simulink model "TestModel_HeliCE150_PID_FFCwithNN"  (R2020b)
settings: Solver=FixedStepAuto  StartTime=0.0  StopTime=Inf  FixedStep=1e-2  RelTol=1e-3
InitFcn:
  | Param_HeliCE150_PID_FFCwithNN
values from neighbouring files (symbols this model uses):
  a_1 = 0.105    [Main_HeliCE150_PID_FFCwithNN.m]    (also in Param_HeliCE150_PID_FFCwithNN.m)
  a_2 = 0.033    [Main_HeliCE150_PID_FFCwithNN.m]    (also in Param_HeliCE150_PID_FFCwithNN.m)
  b_1 = 0.00936    [Main_HeliCE150_PID_FFCwithNN.m]    (also in Param_HeliCE150_PID_FFCwithNN.m)
  b_2 = 0.0294    [Main_HeliCE150_PID_FFCwithNN.m]    (also in Param_HeliCE150_PID_FFCwithNN.m)
  B_phi = 0.00869    [Main_HeliCE150_PID_FFCwithNN.m]    (also in Param_HeliCE150_PID_FFCwithNN.m)
  B_psi = 0.00184    [Main_HeliCE150_PID_FFCwithNN.m]    (also in Param_HeliCE150_PID_FFCwithNN.m)
  I = 0.00437    [Main_HeliCE150_PID_FFCwithNN.m]    (also in Param_HeliCE150_PID_FFCwithNN.m)
  I_phi = 0.00414    [Main_HeliCE150_PID_FFCwithNN.m]    (also in Param_HeliCE150_PID_FFCwithNN.m)
  K_Gyro = 0.015    [Main_HeliCE150_PID_FFCwithNN.m]    (also in Param_HeliCE150_PID_FFCwithNN.m)
  K_r = 0.00162    [Main_HeliCE150_PID_FFCwithNN.m]    (also in Param_HeliCE150_PID_FFCwithNN.m)
  T_0r = 2.7    [Main_HeliCE150_PID_FFCwithNN.m]    (also in Param_HeliCE150_PID_FFCwithNN.m)
  T_1 = 0.3    [Main_HeliCE150_PID_FFCwithNN.m]    (also in Param_HeliCE150_PID_FFCwithNN.m)
  T_2 = 0.25    [Main_HeliCE150_PID_FFCwithNN.m]    (also in Param_HeliCE150_PID_FFCwithNN.m)
  T_pr = 0.75    [Main_HeliCE150_PID_FFCwithNN.m]    (also in Param_HeliCE150_PID_FFCwithNN.m)
  T_u1 = 0    [Main_HeliCE150_PID_FFCwithNN.m]    (also in Param_HeliCE150_PID_FFCwithNN.m)
  T_u2 = 1    [Main_HeliCE150_PID_FFCwithNN.m]    (also in Param_HeliCE150_PID_FFCwithNN.m)
  Tau_g = 0.0383    [Main_HeliCE150_PID_FFCwithNN.m]    (also in Param_HeliCE150_PID_FFCwithNN.m)
libraries: neural x24, pid_lib x3
(part 1 of 2)
settings Model: Creator=Juraj  LastModifiedBy=Juraj

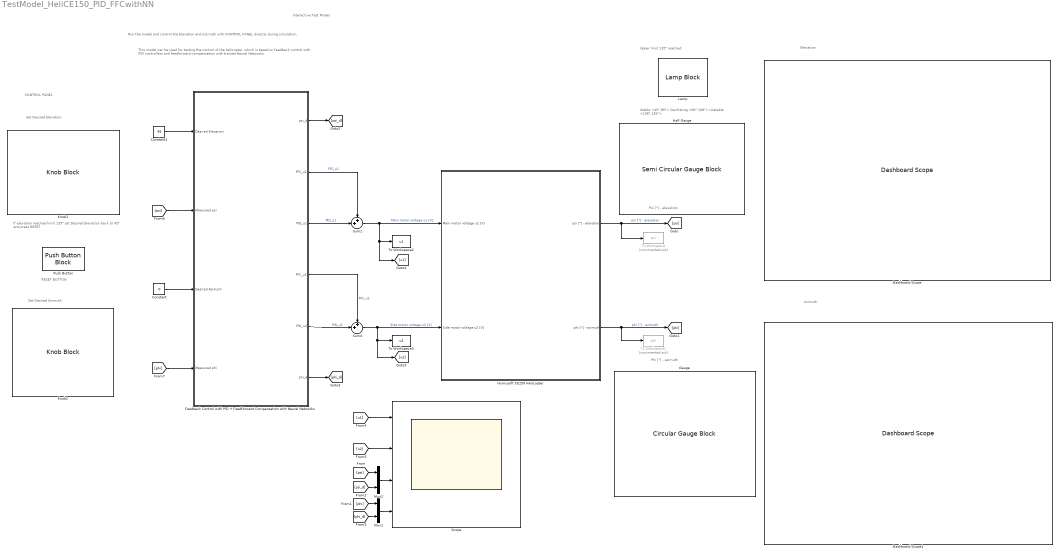
== system TestModel_HeliCE150_PID_FFCwithNN ==
  note: Stable <45°,90°>
      | Oscillating <90°,108°>
      | Unstable <108°,135°>
  note: Run the model and control the Elevation and Azimuth with CONTROL PANEL directly during simulation.
  note: Phi [°] - azimuth
  note: Psi [°] - elevation
  note: Elevation
  note: This model can be used for testing the control of the helicopter, which is based on
      | feedback control with PID controllers and feedforward compensation with trained Neural Networks
  note: Interactive Test Model
  note: CONTROL PANEL
  note: If elevation reached limit 135°
      | set Desired Elevation back to 45° and press RESET
  note: RESET BUTTON
  note: Set Desired Elevation
  note: Set Desired Azimuth
  note: Upper limit 135° reached
  note: Azimuth
  Constant : Constant  Value=0
  Constant1 : Constant  Value=45
  Dashboard Scope : DashboardScope  TimeSpan=1000  Ymin=40  Ymax=140  ScaleAtStop=off
  Dashboard Scope1 : DashboardScope  TimeSpan=1000  Ymin=-140  Ymax=140  ScaleAtStop=off
  Feedback Control with PID + Feedforward Compensation with Neural Networks : Subsystem
  Gauge : CircularGaugeBlock  LabelPosition=Hide  ScaleMin=-130  ScaleMax=130  TickInterval=20
  Half Gauge : SemiCircularGaugeBlock  LabelPosition=Hide  ScaleMin=45  ScaleMax=135  TickInterval=15
  Humusoft CE150 Helicopter : Subsystem
      mask Display: image('$imagefile'); % Use "Edit Image" on toolstrip to change.
  Knob1 : KnobBlock  LabelPosition=Hide  ScaleMin=45  ScaleMax=135  TickInterval=5
  Knob2 : KnobBlock  LabelPosition=Hide  ScaleMin=-130  ScaleMax=130  TickInterval=10
  Lamp : LampBlock  LabelPosition=Hide
  Mux1 : Mux  Inputs=2
  Mux2 : Mux  Inputs=2
  Push Button : PushButtonBlock  ButtonText=RESET
  Scope : Scope  NumInputPorts=4
  Sum1 : Sum  Inputs=++|
  Sum4 : Sum  Inputs=++|
  To Workspace : ToWorkspace  Commented=on  VariableName=psi  SampleTime=-1
  To Workspace1 : ToWorkspace  Commented=on  VariableName=phi  SampleTime=-1
  To Workspace2 : ToWorkspace  VariableName=u1  SampleTime=-1
  To Workspace3 : ToWorkspace  VariableName=u2  SampleTime=-1
  wires:
  [psi] -> Mux2/1
  Sum4/1 -> [u2], To Workspace3/1, Humusoft CE150 Helicopter/2(Side motor voltage u2 [V])  "Side motor voltage u2 [V]"
  Humusoft CE150 Helicopter/1(psi [°] - elevation) -> To Workspace/1, [psi]  "psi [°] - elevation"
  [u1] -> Scope/1
  Humusoft CE150 Helicopter/2(phi [°] - azimuth) -> To Workspace1/1, [phi]  "phi [°] - azimuth"
  [phi] -> Mux1/1
  [psi_d] -> Mux2/2
  Mux1/1 -> Scope/4
  Mux2/1 -> Scope/3
  Sum1/1 -> [u1], To Workspace2/1, Humusoft CE150 Helicopter/1(Main motor voltage u1 [V])  "Main motor voltage u1 [V]"
  [u2] -> Scope/2
  [phi_d] -> Mux1/2
  Feedback Control with PID + Feedforward Compensation with Neural Networks/6(phi_d) -> [phi_d]
  Feedback Control with PID + Feedforward Compensation with Neural Networks/5(PID_u2) -> Sum4/2  "PID_u2"
  Feedback Control with PID + Feedforward Compensation with Neural Networks/2(FFC_u1) -> Sum1/1  "FFC_u1"
  Feedback Control with PID + Feedforward Compensation with Neural Networks/1(psi_d) -> [psi_d]
  [psi] -> Feedback Control with PID + Feedforward Compensation with Neural Networks/2(Measured psi)
  Feedback Control with PID + Feedforward Compensation with Neural Networks/4(FFC_u2) -> Sum4/1  "FFC_u2"
  Feedback Control with PID + Feedforward Compensation with Neural Networks/3(PID_u1) -> Sum1/2  "PID_u1"
  [phi] -> Feedback Control with PID + Feedforward Compensation with Neural Networks/4(Measured phi)
  Constant/1 -> Feedback Control with PID + Feedforward Compensation with Neural Networks/3(Desired Azimuth)
  Constant1/1 -> Feedback Control with PID + Feedforward Compensation with Neural Networks/1(Desired Elevation)

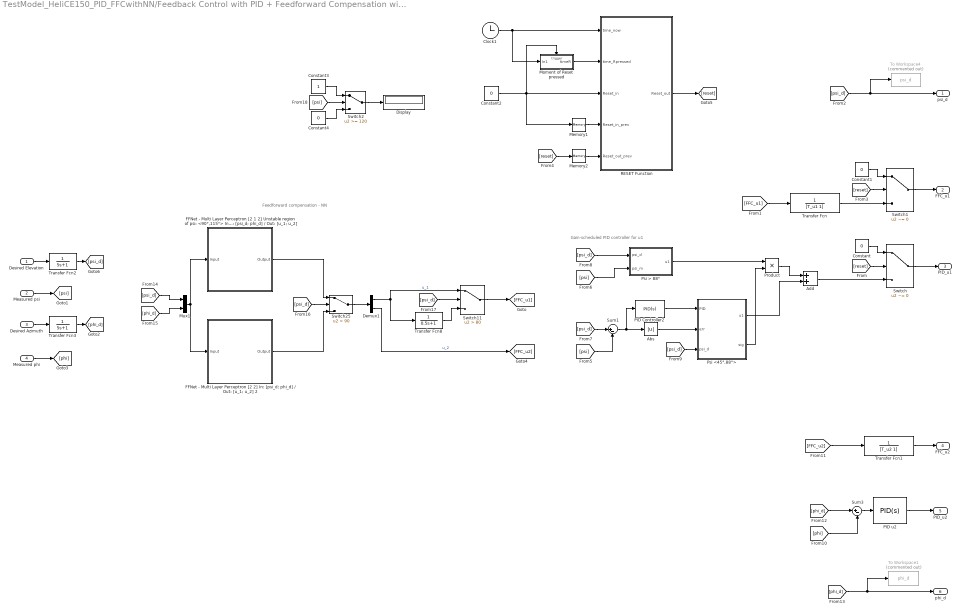
== system TestModel_HeliCE150_PID_FFCwithNN/Feedback Control with PID + Feedforward Compensation with Neural Networks ==
  note: Feedforward compensation - NN
  note: Gain-scheduled PID controller for u1
  Desired Elevation : Inport
  Measured psi : Inport  Port=2
  Desired Azimuth : Inport  Port=3
  Measured phi : Inport  Port=4
  Abs : Abs
  Add : Sum
  Clock1 : Clock
  Constant{,1..2,4} (4 alike) : Constant  Value=0
  Constant3 : Constant
  Demux1 : Demux  Outputs=2
  Display : Display
  FFNet - Multi Layer Perceptron [2 1 2] Unstable region of psi: <90°,115°> In: [psi_d; phi_d] / Out: [u_1; u_2] : Subsystem
      mask help: Feed-Forward Neural Network
      mask Display: e = 0.06;c1 = [120 150 230]/255;c2 = ([120 150 230]+0)/383;c3 = ([120 150 230]+128)/383;patch([0 1 1 0],[0 0 1 1],c1);patch([0 1 1 1-e 1-e 0+e],[0 0 1 1-e 0+e 0+e],c2);patch([0 0 1 1-e 0+e 0+e],[0 1 1 1-e 1-e 0+e],c3);plot([0 1 1 0 0],[0 0 1 1 0]);fprintf('NNET');port_label('input',1,' Input');port_label('output',1,'Output ');
  FFNet - Multi Layer Perceptron [2 2] In: [psi_d; phi_d] / Out: [u_1; u_2] 2 : Subsystem
      mask help: Feed-Forward Neural Network
      mask Display: e = 0.06;c1 = [120 150 230]/255;c2 = ([120 150 230]+0)/383;c3 = ([120 150 230]+128)/383;patch([0 1 1 0],[0 0 1 1],c1);patch([0 1 1 1-e 1-e 0+e],[0 0 1 1-e 0+e 0+e],c2);patch([0 0 1 1-e 0+e 0+e],[0 1 1 1-e 1-e 0+e],c3);plot([0 1 1 0 0],[0 0 1 1 0]);fprintf('NNET');port_label('input',1,' Input');port_label('output',1,'Output ');
  Memory1 : Memory
  Memory2 : Memory
  Moment of Reset pressed : Subsystem  TreatAsAtomicUnit=on
  Mux1 : Mux  Inputs=2
  PID Controller2 : pid_lib/PID Controller  Controller=PID  Form=Parallel  TimeDomain=Continuous-time  UseExternalTs=off  SampleTime=-1  IntegratorMethod=Forward Euler  FilterMethod=Forward Euler  ControllerParametersSource=internal  P=0.001  I=0  D=0.005  UseFilter=on  N=100  TunerSelectOption=Transfer Function Based (PID Tuner App)  InitialConditionSource=internal  InitialConditionForIntegrator=0  InitialConditionForFilter=0  DifferentiatorICPrevScaledInput=0  ExternalReset=none  TrackingMode=off  Kt=1  LimitOutput=on  SatLimitsSource=internal  UpperSaturationLimit=1  LowerSaturationLimit=-1  LinearizeAsGain=on  AntiWindupMode=clamping  Kb=1  POutMin=[]  POutMax=[]  IOutMin=[]  IOutMax=[]  DOutMin=[]  DOutMax=[]  NOutMin=[]  NOutMax=[]  SumOutMin=[]  SumOutMax=[]  SaturationOutMin=[]  SaturationOutMax=[]  PParamMin=[]  PParamMax=[]  IParamMin=[]  IParamMax=[]  DParamMin=[]  DParamMax=[]  NParamMin=[]  NParamMax=[]  KbParamMin=[]  KbParamMax=[]  KtParamMin=[]  KtParamMax=[]  KbOutMin=[]  KbOutMax=[]  KtOutMin=[]  KtOutMax=[]  IntegratorOutMin=[]  IntegratorOutMax=[]  FilterOutMin=[]  FilterOutMax=[]  SumI1OutMin=[]  SumI1OutMax=[]  SumI2OutMin=[]  SumI2OutMax=[]  SumI3OutMin=[]  SumI3OutMax=[]  SumI4OutMin=[]  SumI4OutMax=[]  SumDOutMin=[]  SumDOutMax=[]  DifferentiatorOutMin=[]  DifferentiatorOutMax=[]  FilterDiffOutCoefMin=[]  FilterDiffOutCoefMax=[]  ReciprocalOutMin=[]  ReciprocalOutMax=[]  SumDenOutMin=[]  SumDenOutMax=[]  SumNumOutMin=[]  SumNumOutMax=[]  DivideOutMin=[]  DivideOutMax=[]  UdiffTsProdOutMin=[]  UdiffTsProdOutMax=[]  NTsProdOutMin=[]  NTsProdOutMax=[]  UintegralTsProdOutMin=[]  UintegralTsProdOutMax=[]  UngainTsProdOutMin=[]  UngainTsProdOutMax=[]  IntegratorContinuousStateAttributes=''  IntegratorStateMustResolveToSignalObject=off  IntegratorRTWStateStorageClass=Auto  FilterContinuousStateAttributes=''  FilterStateMustResolveToSignalObject=off  FilterRTWStateStorageClass=Auto  ParallelPVariant=InternalParameters  IdealPVariant=Disabled  IVariant=InternalParameters  DVariant=InternalParameters  IntegratorVariant=Continuous  SatVariant=Enabled  AWVariant=ContClampingParallel  PCopyVariant=Disabled  TRVariant=Disabled  FdbkBlocksVariant=Forward  IdealPFdbkVariant=Disabled  SatFdbkVariant=Disabled  DerivativeFilterVariant=ContFilter  NVariant=InternalParameters  NCopyVariant=Disabled  FilterICVariant=InternalICsFilter  IntegratorICVariant=InternalICs  ExternalResetVariant=Disabled  TRSumVariant=Passthrough  SumFdbkVariant=Disabled  SumVariant=Sum_PID  TsampFilterVariant=InternalTs  TsampNgainVariant=Passthrough  TsampIntegralVariant=Passthrough  ExternalSaturationOutDataTypeStr=Inherit: Same as second input
  PID u2 : pid_lib/PID Controller  Controller=PID  Form=Parallel  TimeDomain=Continuous-time  UseExternalTs=off  SampleTime=-1  IntegratorMethod=Forward Euler  FilterMethod=Forward Euler  ControllerParametersSource=internal  P=0.01  I=0  D=0.01  UseFilter=on  N=100  TunerSelectOption=Transfer Function Based (PID Tuner App)  InitialConditionSource=internal  InitialConditionForIntegrator=0  InitialConditionForFilter=0  DifferentiatorICPrevScaledInput=0  ExternalReset=none  TrackingMode=off  Kt=1  LimitOutput=on  SatLimitsSource=internal  UpperSaturationLimit=1  LowerSaturationLimit=-1  LinearizeAsGain=on  AntiWindupMode=none  Kb=1  POutMin=[]  POutMax=[]  IOutMin=[]  IOutMax=[]  DOutMin=[]  DOutMax=[]  NOutMin=[]  NOutMax=[]  SumOutMin=[]  SumOutMax=[]  SaturationOutMin=[]  SaturationOutMax=[]  PParamMin=[]  PParamMax=[]  IParamMin=[]  IParamMax=[]  DParamMin=[]  DParamMax=[]  NParamMin=[]  NParamMax=[]  KbParamMin=[]  KbParamMax=[]  KtParamMin=[]  KtParamMax=[]  KbOutMin=[]  KbOutMax=[]  KtOutMin=[]  KtOutMax=[]  IntegratorOutMin=[]  IntegratorOutMax=[]  FilterOutMin=[]  FilterOutMax=[]  SumI1OutMin=[]  SumI1OutMax=[]  SumI2OutMin=[]  SumI2OutMax=[]  SumI3OutMin=[]  SumI3OutMax=[]  SumI4OutMin=[]  SumI4OutMax=[]  SumDOutMin=[]  SumDOutMax=[]  DifferentiatorOutMin=[]  DifferentiatorOutMax=[]  FilterDiffOutCoefMin=[]  FilterDiffOutCoefMax=[]  ReciprocalOutMin=[]  ReciprocalOutMax=[]  SumDenOutMin=[]  SumDenOutMax=[]  SumNumOutMin=[]  SumNumOutMax=[]  DivideOutMin=[]  DivideOutMax=[]  UdiffTsProdOutMin=[]  UdiffTsProdOutMax=[]  NTsProdOutMin=[]  NTsProdOutMax=[]  UintegralTsProdOutMin=[]  UintegralTsProdOutMax=[]  UngainTsProdOutMin=[]  UngainTsProdOutMax=[]  IntegratorContinuousStateAttributes=''  IntegratorStateMustResolveToSignalObject=off  IntegratorRTWStateStorageClass=Auto  FilterContinuousStateAttributes=''  FilterStateMustResolveToSignalObject=off  FilterRTWStateStorageClass=Auto  ParallelPVariant=InternalParameters  IdealPVariant=Disabled  IVariant=InternalParameters  DVariant=InternalParameters  IntegratorVariant=Continuous  SatVariant=Enabled  AWVariant=Passthrough  PCopyVariant=Disabled  TRVariant=Disabled  FdbkBlocksVariant=Forward  IdealPFdbkVariant=Disabled  SatFdbkVariant=Disabled  DerivativeFilterVariant=ContFilter  NVariant=InternalParameters  NCopyVariant=Disabled  FilterICVariant=InternalICsFilter  IntegratorICVariant=InternalICs  ExternalResetVariant=Disabled  TRSumVariant=Passthrough  SumFdbkVariant=Disabled  SumVariant=Sum_PID  TsampFilterVariant=InternalTs  TsampNgainVariant=Passthrough  TsampIntegralVariant=Passthrough  ExternalSaturationOutDataTypeStr=Inherit: Same as second input
  Product : Product
  Psi <45°,88°> : MATLAB Function  TreatAsAtomicUnit=on
  Psi > 88° : Subsystem
  RESET Function : MATLAB Function  TreatAsAtomicUnit=on
  Sum1 : Sum  Inputs=|+-
  Sum3 : Sum  Inputs=|+-
  Switch : Switch  Criteria=u2 ~= 0
  Switch1 : Switch  Criteria=u2 ~= 0
  Switch11 : Switch  Criteria=u2 > Threshold  Threshold=80
  Switch2 : Switch  Threshold=120
  Switch25 : Switch  Criteria=u2 > Threshold  Threshold=90
  To Workspace1 : ToWorkspace  Commented=on  VariableName=phi_d  SampleTime=-1
  To Workspace4 : ToWorkspace  Commented=on  VariableName=psi_d  SampleTime=-1
  Transfer Fcn : TransferFcn  Denominator=[T_u1 1]
  Transfer Fcn1 : TransferFcn  Denominator=[T_u2 1]
  Transfer Fcn2 : TransferFcn  Denominator=[5 1]
  Transfer Fcn3 : TransferFcn  Denominator=[5 1]
  Transfer Fcn8 : TransferFcn  Denominator=[0.5 1]
  psi_d : Outport
  FFC_u1 : Outport  Port=2
  PID_u1 : Outport  Port=3
  FFC_u2 : Outport  Port=4
  PID_u2 : Outport  Port=5
  phi_d : Outport  Port=6
  wires:
  Sum3/1 -> PID u2/1
  Transfer Fcn/1 -> Switch1/3
  [FFC_u1] -> Transfer Fcn/1
  [psi_d] -> To Workspace4/1, psi_d/1
  Measured psi/1 -> [psi]
  Measured phi/1 -> [phi]
  Add/1 -> Switch/3
  Product/1 -> Add/1
  Psi <45°,88°>/1(u1) -> Add/2
  [psi_d] -> Psi <45°,88°>/3(psi_d)
  PID Controller2/1 -> Psi <45°,88°>/1(PID)
  Psi <45°,88°>/2(sig) -> Product/2
  [psi] -> Psi > 88°/2(psi_m)
  Psi > 88°/1(u1) -> Product/1
  [psi_d] -> Psi > 88°/1(psi_d)
  Sum1/1 -> Abs/1, PID Controller2/1
  [psi_d] -> Sum1/1
  [psi] -> Sum1/2
  Abs/1 -> Psi <45°,88°>/2(err)
  [FFC_u2] -> Transfer Fcn1/1
  Transfer Fcn1/1 -> FFC_u2/1
  [phi_d] -> Sum3/1
  [phi] -> Sum3/2
  PID u2/1 -> PID_u2/1
  [phi_d] -> phi_d/1, To Workspace1/1
  [psi_d] -> Switch25/2
  FFNet - Multi Layer Perceptron [2 2] In: [psi_d; phi_d] / Out: [u_1; u_2] 2/1(Output) -> Switch25/3
  FFNet - Multi Layer Perceptron [2 1 2] Unstable region of psi: <90°,115°> In: [psi_d; phi_d] / Out: [u_1; u_2]/1(Output) -> Switch25/1
  Switch11/1 -> [FFC_u1]
  [phi_d] -> Mux1/2
  [psi_d] -> Mux1/1
  Demux1/1 -> Transfer Fcn8/1, Switch11/1  "u_1"
  Mux1/1 -> FFNet - Multi Layer Perceptron [2 2] In: [psi_d; phi_d] / Out: [u_1; u_2] 2/1(Input), FFNet - Multi Layer Perceptron [2 1 2] Unstable region of psi: <90°,115°> In: [psi_d; phi_d] / Out: [u_1; u_2]/1(Input)
  Transfer Fcn8/1 -> Switch11/3
  [psi_d] -> Switch11/2
  Switch25/1 -> Demux1/1
  Demux1/2 -> [FFC_u2]  "u_2"
  Desired Elevation/1 -> Transfer Fcn2/1
  Desired Azimuth/1 -> Transfer Fcn3/1
  Transfer Fcn2/1 -> [psi_d]
  Transfer Fcn3/1 -> [phi_d]
  [reset] -> Switch/2
  Switch/1 -> PID_u1/1
  Constant/1 -> Switch/1
  [reset] -> Switch1/2
  Constant1/1 -> Switch1/1
  Switch1/1 -> FFC_u1/1
  RESET Function/1(Reset_out) -> [reset]
  Memory1/1 -> RESET Function/4(Reset_in_prev)
  Clock1/1 -> Moment of Reset pressed/1(In1), RESET Function/1(time_now)
  Constant2/1 -> RESET Function/3(Reset_in), Memory1/1, Moment of Reset pressed/Trigger
  Moment of Reset pressed/1(timeR) -> RESET Function/2(time_Rpressed)
  Memory2/1 -> RESET Function/5(Reset_out_prev)
  [reset] -> Memory2/1
  [psi] -> Switch2/2
  Constant4/1 -> Switch2/3
  Constant3/1 -> Switch2/1
  Switch2/1 -> Display/1

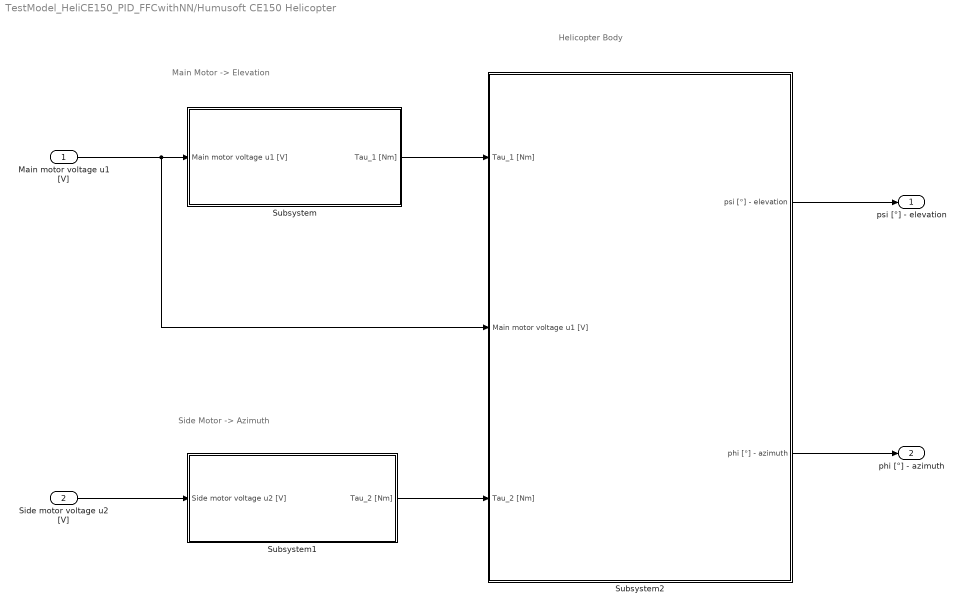
== system TestModel_HeliCE150_PID_FFCwithNN/Humusoft CE150 Helicopter ==
  note: Helicopter Body
  note: Side Motor -> Azimuth
  note: Main Motor -> Elevation
  Main motor voltage u1 [V] : Inport
  Side motor voltage u2 [V] : Inport  Port=2
  Subsystem : Subsystem
  Subsystem1 : Subsystem
  Subsystem2 : Subsystem
  psi [°] - elevation : Outport
  phi [°] - azimuth : Outport  Port=2
  wires:
  Main motor voltage u1 [V]/1 -> Subsystem2/2(Main motor voltage u1 [V]), Subsystem/1(Main motor voltage u1 [V])
  Side motor voltage u2 [V]/1 -> Subsystem1/1(Side motor voltage u2 [V])
  Subsystem/1(Tau_1 [Nm]) -> Subsystem2/1(Tau_1 [Nm])
  Subsystem1/1(Tau_2 [Nm]) -> Subsystem2/3(Tau_2 [Nm])
  Subsystem2/1(psi [°] - elevation) -> psi [°] - elevation/1
  Subsystem2/2(phi [°] - azimuth) -> phi [°] - azimuth/1

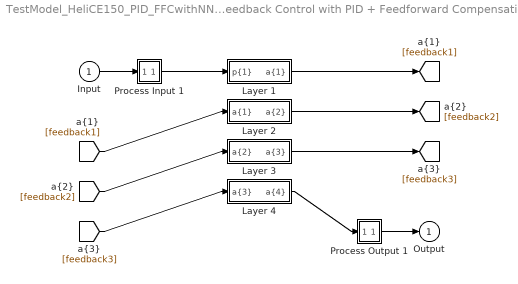
== system TestModel_HeliCE150_PID_FFCwithNN/Feedback Control with PID + Feedforward Compensation with Neural Networks/FFNet - Multi Layer Perceptron [2 1 2] Unstable region of psi: <90°,115°> In: [psi_d; phi_d] // Out: [u_1; u_2] ==
  Input : Inport  PortDimensions=2
      mask Display: e = 0.06;c1 = [120 230 180]/255;c2 = ([120 230 180]+0)/(256+128);c3 = ([120 230 180]+128)/(256+128);patch([0 1 1 0],[0 0 1 1],c1);patch([0 1 1 1-e 1-e 0+e],[0 0 1 1-e 0+e 0+e],c2);patch([0 0 1 1-e 0+e 0+e],[0 1 1 1-e 1-e 0+e],c3);plot([0 1 1 0 0],[0 0 1 1 0]);
  Layer 1 : Subsystem
      mask Display: e = 0.06;c1 = [120 150 230]/255;c2 = ([120 150 230]+0)/383;c3 = ([120 150 230]+128)/383;patch([0 1 1 0],[0 0 1 1],c1);patch([0 1 1 1-e 1-e 0+e],[0 0 1 1-e 0+e 0+e],c2);patch([0 0 1 1-e 0+e 0+e],[0 1 1 1-e 1-e 0+e],c3);plot([0 1 1 0 0],[0 0 1 1 0]);
  Layer 2 : Subsystem
      mask Display: e = 0.06;c1 = [120 150 230]/255;c2 = ([120 150 230]+0)/383;c3 = ([120 150 230]+128)/383;patch([0 1 1 0],[0 0 1 1],c1);patch([0 1 1 1-e 1-e 0+e],[0 0 1 1-e 0+e 0+e],c2);patch([0 0 1 1-e 0+e 0+e],[0 1 1 1-e 1-e 0+e],c3);plot([0 1 1 0 0],[0 0 1 1 0]);
  Layer 3 : Subsystem
      mask Display: e = 0.06;c1 = [120 150 230]/255;c2 = ([120 150 230]+0)/383;c3 = ([120 150 230]+128)/383;patch([0 1 1 0],[0 0 1 1],c1);patch([0 1 1 1-e 1-e 0+e],[0 0 1 1-e 0+e 0+e],c2);patch([0 0 1 1-e 0+e 0+e],[0 1 1 1-e 1-e 0+e],c3);plot([0 1 1 0 0],[0 0 1 1 0]);
  Layer 4 : Subsystem
      mask Display: e = 0.06;c1 = [120 150 230]/255;c2 = ([120 150 230]+0)/383;c3 = ([120 150 230]+128)/383;patch([0 1 1 0],[0 0 1 1],c1);patch([0 1 1 1-e 1-e 0+e],[0 0 1 1-e 0+e 0+e],c2);patch([0 0 1 1-e 0+e 0+e],[0 1 1 1-e 1-e 0+e],c3);plot([0 1 1 0 0],[0 0 1 1 0]);
  Process Input 1 : Subsystem
      mask Display: e = 0.06;c1 = [120 150 230]/255;c2 = ([120 150 230]+0)/383;c3 = ([120 150 230]+128)/383;patch([0 1 1 0],[0 0 1 1],c1);patch([0 1 1 1-e 1-e 0+e],[0 0 1 1-e 0+e 0+e],c2);patch([0 0 1 1-e 0+e 0+e],[0 1 1 1-e 1-e 0+e],c3);plot([0 1 1 0 0],[0 0 1 1 0]);
  Process Output 1 : Subsystem
      mask Display: e = 0.06;c1 = [120 150 230]/255;c2 = ([120 150 230]+0)/383;c3 = ([120 150 230]+128)/383;patch([0 1 1 0],[0 0 1 1],c1);patch([0 1 1 1-e 1-e 0+e],[0 0 1 1-e 0+e 0+e],c2);patch([0 0 1 1-e 0+e 0+e],[0 1 1 1-e 1-e 0+e],c3);plot([0 1 1 0 0],[0 0 1 1 0]);
  Output : Outport  InitialOutput=[0;0]
      mask Display: e = 0.06;c1 = [120 230 180]/255;c2 = ([120 230 180]+0)/(256+128);c3 = ([120 230 180]+128)/(256+128);patch([0 1 1 0],[0 0 1 1],c1);patch([0 1 1 1-e 1-e 0+e],[0 0 1 1-e 0+e 0+e],c2);patch([0 0 1 1-e 0+e 0+e],[0 1 1 1-e 1-e 0+e],c3);plot([0 1 1 0 0],[0 0 1 1 0]);
  wires:
  Input/1 -> Process Input 1/1(x)
  Process Output 1/1(y) -> Output/1
  Process Input 1/1(p) -> Layer 1/1("p{1}")
  Layer 1/1("a{1}") -> [feedback1]
  [feedback1] -> Layer 2/1("a{1} ")
  Layer 2/1("a{2}") -> [feedback2]
  [feedback2] -> Layer 3/1("a{2} ")
  Layer 3/1("a{3}") -> [feedback3]
  [feedback3] -> Layer 4/1("a{3} ")
  Layer 4/1("a{4}") -> Process Output 1/1(a)

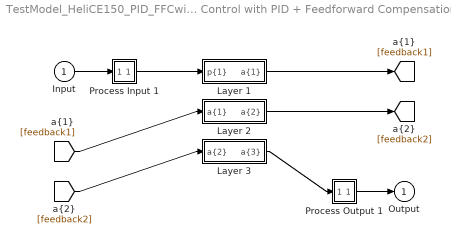
== system TestModel_HeliCE150_PID_FFCwithNN/Feedback Control with PID + Feedforward Compensation with Neural Networks/FFNet - Multi Layer Perceptron [2 2] In: [psi_d; phi_d] // Out: [u_1; u_2] 2 ==
  Input : Inport  PortDimensions=2
      mask Display: e = 0.06;c1 = [120 230 180]/255;c2 = ([120 230 180]+0)/(256+128);c3 = ([120 230 180]+128)/(256+128);patch([0 1 1 0],[0 0 1 1],c1);patch([0 1 1 1-e 1-e 0+e],[0 0 1 1-e 0+e 0+e],c2);patch([0 0 1 1-e 0+e 0+e],[0 1 1 1-e 1-e 0+e],c3);plot([0 1 1 0 0],[0 0 1 1 0]);
  Layer 1 : Subsystem
      mask Display: e = 0.06;c1 = [120 150 230]/255;c2 = ([120 150 230]+0)/383;c3 = ([120 150 230]+128)/383;patch([0 1 1 0],[0 0 1 1],c1);patch([0 1 1 1-e 1-e 0+e],[0 0 1 1-e 0+e 0+e],c2);patch([0 0 1 1-e 0+e 0+e],[0 1 1 1-e 1-e 0+e],c3);plot([0 1 1 0 0],[0 0 1 1 0]);
  Layer 2 : Subsystem
      mask Display: e = 0.06;c1 = [120 150 230]/255;c2 = ([120 150 230]+0)/383;c3 = ([120 150 230]+128)/383;patch([0 1 1 0],[0 0 1 1],c1);patch([0 1 1 1-e 1-e 0+e],[0 0 1 1-e 0+e 0+e],c2);patch([0 0 1 1-e 0+e 0+e],[0 1 1 1-e 1-e 0+e],c3);plot([0 1 1 0 0],[0 0 1 1 0]);
  Layer 3 : Subsystem
      mask Display: e = 0.06;c1 = [120 150 230]/255;c2 = ([120 150 230]+0)/383;c3 = ([120 150 230]+128)/383;patch([0 1 1 0],[0 0 1 1],c1);patch([0 1 1 1-e 1-e 0+e],[0 0 1 1-e 0+e 0+e],c2);patch([0 0 1 1-e 0+e 0+e],[0 1 1 1-e 1-e 0+e],c3);plot([0 1 1 0 0],[0 0 1 1 0]);
  Process Input 1 : Subsystem
      mask Display: e = 0.06;c1 = [120 150 230]/255;c2 = ([120 150 230]+0)/383;c3 = ([120 150 230]+128)/383;patch([0 1 1 0],[0 0 1 1],c1);patch([0 1 1 1-e 1-e 0+e],[0 0 1 1-e 0+e 0+e],c2);patch([0 0 1 1-e 0+e 0+e],[0 1 1 1-e 1-e 0+e],c3);plot([0 1 1 0 0],[0 0 1 1 0]);
  Process Output 1 : Subsystem
      mask Display: e = 0.06;c1 = [120 150 230]/255;c2 = ([120 150 230]+0)/383;c3 = ([120 150 230]+128)/383;patch([0 1 1 0],[0 0 1 1],c1);patch([0 1 1 1-e 1-e 0+e],[0 0 1 1-e 0+e 0+e],c2);patch([0 0 1 1-e 0+e 0+e],[0 1 1 1-e 1-e 0+e],c3);plot([0 1 1 0 0],[0 0 1 1 0]);
  Output : Outport  InitialOutput=[0;0]
      mask Display: e = 0.06;c1 = [120 230 180]/255;c2 = ([120 230 180]+0)/(256+128);c3 = ([120 230 180]+128)/(256+128);patch([0 1 1 0],[0 0 1 1],c1);patch([0 1 1 1-e 1-e 0+e],[0 0 1 1-e 0+e 0+e],c2);patch([0 0 1 1-e 0+e 0+e],[0 1 1 1-e 1-e 0+e],c3);plot([0 1 1 0 0],[0 0 1 1 0]);
  wires:
  Layer 3/1("a{3}") -> Process Output 1/1(a)
  [feedback2] -> Layer 3/1("a{2} ")
  Layer 2/1("a{2}") -> [feedback2]
  [feedback1] -> Layer 2/1("a{1} ")
  Layer 1/1("a{1}") -> [feedback1]
  Process Input 1/1(p) -> Layer 1/1("p{1}")
  Process Output 1/1(y) -> Output/1
  Input/1 -> Process Input 1/1(x)

== system TestModel_HeliCE150_PID_FFCwithNN/Feedback Control with PID + Feedforward Compensation with Neural Networks/Moment of Reset pressed ==
  In1 : Inport
  Trigger : TriggerPort  VariantControl=(inherit)
  timeR : Outport
  wires:
  In1/1 -> timeR/1

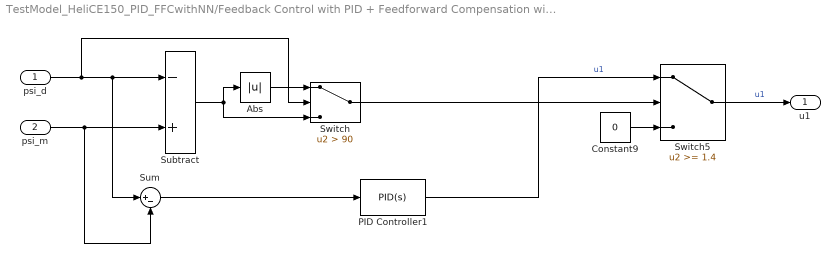
== system TestModel_HeliCE150_PID_FFCwithNN/Feedback Control with PID + Feedforward Compensation with Neural Networks/Psi > 88° ==
  psi_d : Inport
  psi_m : Inport  Port=2
  Abs : Abs
  Constant9 : Constant  Value=0
  PID Controller1 : pid_lib/PID Controller  Controller=PID  Form=Parallel  TimeDomain=Continuous-time  UseExternalTs=off  SampleTime=-1  IntegratorMethod=Forward Euler  FilterMethod=Forward Euler  ControllerParametersSource=internal  P=0.0001  I=0  D=0.015  UseFilter=on  N=100  TunerSelectOption=Transfer Function Based (PID Tuner App)  InitialConditionSource=internal  InitialConditionForIntegrator=0  InitialConditionForFilter=0  DifferentiatorICPrevScaledInput=0  ExternalReset=none  TrackingMode=off  Kt=1  LimitOutput=on  SatLimitsSource=internal  UpperSaturationLimit=1  LowerSaturationLimit=-1  LinearizeAsGain=on  AntiWindupMode=clamping  Kb=1  POutMin=[]  POutMax=[]  IOutMin=[]  IOutMax=[]  DOutMin=[]  DOutMax=[]  NOutMin=[]  NOutMax=[]  SumOutMin=[]  SumOutMax=[]  SaturationOutMin=[]  SaturationOutMax=[]  PParamMin=[]  PParamMax=[]  IParamMin=[]  IParamMax=[]  DParamMin=[]  DParamMax=[]  NParamMin=[]  NParamMax=[]  KbParamMin=[]  KbParamMax=[]  KtParamMin=[]  KtParamMax=[]  KbOutMin=[]  KbOutMax=[]  KtOutMin=[]  KtOutMax=[]  IntegratorOutMin=[]  IntegratorOutMax=[]  FilterOutMin=[]  FilterOutMax=[]  SumI1OutMin=[]  SumI1OutMax=[]  SumI2OutMin=[]  SumI2OutMax=[]  SumI3OutMin=[]  SumI3OutMax=[]  SumI4OutMin=[]  SumI4OutMax=[]  SumDOutMin=[]  SumDOutMax=[]  DifferentiatorOutMin=[]  DifferentiatorOutMax=[]  FilterDiffOutCoefMin=[]  FilterDiffOutCoefMax=[]  ReciprocalOutMin=[]  ReciprocalOutMax=[]  SumDenOutMin=[]  SumDenOutMax=[]  SumNumOutMin=[]  SumNumOutMax=[]  DivideOutMin=[]  DivideOutMax=[]  UdiffTsProdOutMin=[]  UdiffTsProdOutMax=[]  NTsProdOutMin=[]  NTsProdOutMax=[]  UintegralTsProdOutMin=[]  UintegralTsProdOutMax=[]  UngainTsProdOutMin=[]  UngainTsProdOutMax=[]  IntegratorContinuousStateAttributes=''  IntegratorStateMustResolveToSignalObject=off  IntegratorRTWStateStorageClass=Auto  FilterContinuousStateAttributes=''  FilterStateMustResolveToSignalObject=off  FilterRTWStateStorageClass=Auto  ParallelPVariant=InternalParameters  IdealPVariant=Disabled  IVariant=InternalParameters  DVariant=InternalParameters  IntegratorVariant=Continuous  SatVariant=Enabled  AWVariant=ContClampingParallel  PCopyVariant=Disabled  TRVariant=Disabled  FdbkBlocksVariant=Forward  IdealPFdbkVariant=Disabled  SatFdbkVariant=Disabled  DerivativeFilterVariant=ContFilter  NVariant=InternalParameters  NCopyVariant=Disabled  FilterICVariant=InternalICsFilter  IntegratorICVariant=InternalICs  ExternalResetVariant=Disabled  TRSumVariant=Passthrough  SumFdbkVariant=Disabled  SumVariant=Sum_PID  TsampFilterVariant=InternalTs  TsampNgainVariant=Passthrough  TsampIntegralVariant=Passthrough  ExternalSaturationOutDataTypeStr=Inherit: Same as second input
  Subtract : Sum  Inputs=-+
  Sum : Sum  Inputs=|+-
  Switch : Switch  Criteria=u2 > Threshold  Threshold=90
  Switch5 : Switch  Threshold=1.4
  u1 : Outport
  wires:
  Constant9/1 -> Switch5/3
  psi_d/1 -> Switch/2, Sum/1, Subtract/1
  Switch5/1 -> u1/1  "u1"
  psi_m/1 -> Sum/2, Subtract/2
  Sum/1 -> PID Controller1/1
  Subtract/1 -> Abs/1, Switch/3
  Switch/1 -> Switch5/2
  Abs/1 -> Switch/1
  PID Controller1/1 -> Switch5/1  "u1"

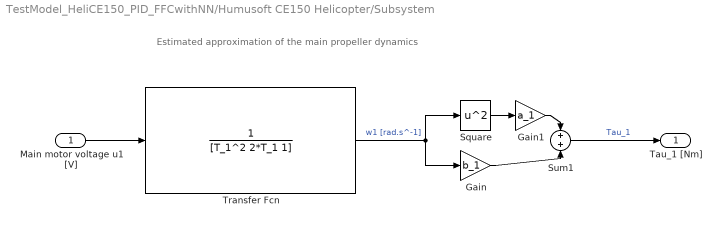
== system TestModel_HeliCE150_PID_FFCwithNN/Humusoft CE150 Helicopter/Subsystem ==
  note: Estimated approximation of the main propeller dynamics
  Main motor voltage u1 [V] : Inport
  Gain : Gain  Gain=b_1
  Gain1 : Gain  Gain=a_1
  Square : Math  Operator=square  SaturateOnIntegerOverflow=on
  Sum1 : Sum  Inputs=+|+
  Transfer Fcn : TransferFcn  Denominator=[T_1^2 2*T_1 1]
  Tau_1 [Nm] : Outport
  wires:
  Gain1/1 -> Sum1/1
  Transfer Fcn/1 -> Gain/1, Square/1  "w1 [rad.s^-1]"
  Square/1 -> Gain1/1
  Gain/1 -> Sum1/2
  Sum1/1 -> Tau_1 [Nm]/1  "Tau_1"
  Main motor voltage u1 [V]/1 -> Transfer Fcn/1

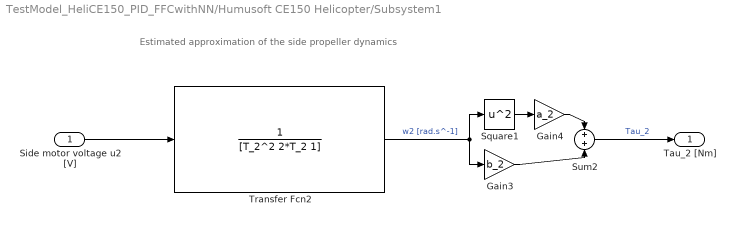
== system TestModel_HeliCE150_PID_FFCwithNN/Humusoft CE150 Helicopter/Subsystem1 ==
  note: Estimated approximation of the side propeller dynamics
  Side motor voltage u2 [V] : Inport
  Gain3 : Gain  Gain=b_2
  Gain4 : Gain  Gain=a_2
  Square1 : Math  Operator=square  SaturateOnIntegerOverflow=on
  Sum2 : Sum  Inputs=+|+
  Transfer Fcn2 : TransferFcn  Denominator=[T_2^2 2*T_2 1]
  Tau_2 [Nm] : Outport
  wires:
  Gain4/1 -> Sum2/1
  Gain3/1 -> Sum2/2
  Sum2/1 -> Tau_2 [Nm]/1  "Tau_2"
  Transfer Fcn2/1 -> Gain3/1, Square1/1  "w2 [rad.s^-1]"
  Side motor voltage u2 [V]/1 -> Transfer Fcn2/1
  Square1/1 -> Gain4/1

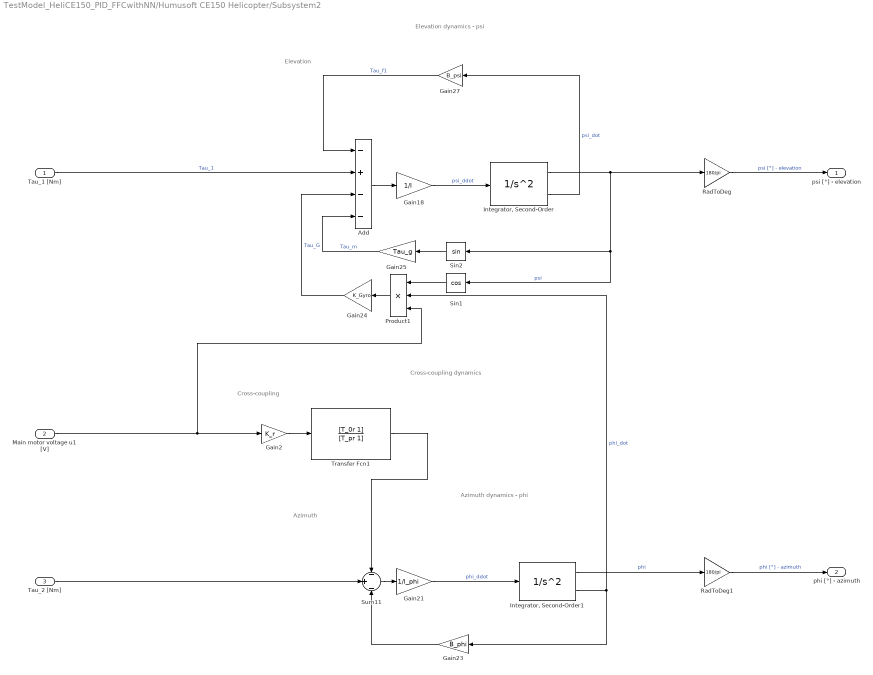
== system TestModel_HeliCE150_PID_FFCwithNN/Humusoft CE150 Helicopter/Subsystem2 ==
  note: Cross-coupling dynamics
  note: Cross-coupling
  note: Azimuth
  note: Elevation
  note: Elevation dynamics - psi
  note: Azimuth dynamics - phi
  Tau_1 [Nm] : Inport
  Main motor voltage u1 [V] : Inport  Port=2
  Tau_2 [Nm] : Inport  Port=3
  Add : Sum  Inputs=-+--
  Gain18 : Gain  Gain=1/I
  Gain2 : Gain  Gain=K_r
  Gain21 : Gain  Gain=1/I_phi
  Gain23 : Gain  Gain=B_phi
  Gain24 : Gain  Gain=K_Gyro
  Gain25 : Gain  Gain=Tau_g
  Gain27 : Gain  Gain=B_psi
  "Integrator, Second-Order" : SecondOrderIntegrator  ICX=pi/4  LimitX=on  UpperLimitX=3*pi/4  LowerLimitX=pi/4
  "Integrator, Second-Order1" : SecondOrderIntegrator  ICX=0*pi/180  LimitX=on  UpperLimitX=130*pi/180  LowerLimitX=-130*pi/180
  Product1 : Product  Inputs=3
  RadToDeg : Gain  Gain=180/pi
  RadToDeg1 : Gain  Gain=180/pi
  Sin1 : Trigonometry  Operator=cos
  Sin2 : Trigonometry
  Sum11 : Sum  Inputs=-|+|-
  Transfer Fcn1 : TransferFcn  Numerator=[T_0r 1]  Denominator=[T_pr 1]
  psi [°] - elevation : Outport
  phi [°] - azimuth : Outport  Port=2
  wires:
  RadToDeg/1 -> psi [°] - elevation/1  "psi [°] - elevation"
  Gain24/1 -> Add/3  "Tau_G"
  "Integrator, Second-Order1"/2 -> Gain23/1, Product1/2  "phi_dot"
  Gain25/1 -> Add/4  "Tau_m"
  Gain27/1 -> Add/1  "Tau_f1"
  Product1/1 -> Gain24/1
  Sin1/1 -> Product1/1
  "Integrator, Second-Order"/2 -> Gain27/1  "psi_dot"
  Gain21/1 -> "Integrator, Second-Order1"/1  "phi_ddot"
  "Integrator, Second-Order"/1 -> Sin1/1, Sin2/1, RadToDeg/1  "psi"
  "Integrator, Second-Order1"/1 -> RadToDeg1/1  "phi"
  Sin2/1 -> Gain25/1
  Tau_2 [Nm]/1 -> Sum11/2
  Gain23/1 -> Sum11/3
  Gain18/1 -> "Integrator, Second-Order"/1  "psi_ddot"
  Sum11/1 -> Gain21/1
  Add/1 -> Gain18/1
  Tau_1 [Nm]/1 -> Add/2  "Tau_1"
  RadToDeg1/1 -> phi [°] - azimuth/1  "phi [°] - azimuth"
  Transfer Fcn1/1 -> Sum11/1
  Main motor voltage u1 [V]/1 -> Product1/3, Gain2/1
  Gain2/1 -> Transfer Fcn1/1

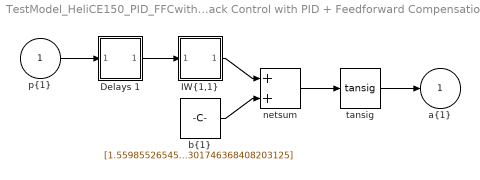
== system TestModel_HeliCE150_PID_FFCwithNN/Feedback Control with PID + Feedforward Compensation with Neural Networks/FFNet - Multi Layer Perceptron [2 1 2] Unstable region of psi: <90°,115°> In: [psi_d; phi_d] // Out: [u_1; u_2]/Layer 1 ==
  "p{1}" : Inport  PortDimensions=2
      mask Display: e = 0.06;c1 = [120 230 180]/255;c2 = ([120 230 180]+0)/(256+128);c3 = ([120 230 180]+128)/(256+128);patch([0 1 1 0],[0 0 1 1],c1);patch([0 1 1 1-e 1-e 0+e],[0 0 1 1-e 0+e 0+e],c2);patch([0 0 1 1-e 0+e 0+e],[0 1 1 1-e 1-e 0+e],c3);plot([0 1 1 0 0],[0 0 1 1 0]);
  Delays 1 : Subsystem
      mask Display: e = 0.06;c1 = [120 150 230]/255;c2 = ([120 150 230]+0)/383;c3 = ([120 150 230]+128)/383;patch([0 1 1 0],[0 0 1 1],c1);patch([0 1 1 1-e 1-e 0+e],[0 0 1 1-e 0+e 0+e],c2);patch([0 0 1 1-e 0+e 0+e],[0 1 1 1-e 1-e 0+e],c3);plot([0 1 1 0 0],[0 0 1 1 0]);disp('0');
  "IW{1,1}" : Subsystem
      mask Display: e = 0.06;c1 = [120 150 230]/255;c2 = ([120 150 230]+0)/383;c3 = ([120 150 230]+128)/383;patch([0 1 1 0],[0 0 1 1],c1);patch([0 1 1 1-e 1-e 0+e],[0 0 1 1-e 0+e 0+e],c2);patch([0 0 1 1-e 0+e 0+e],[0 1 1 1-e 1-e 0+e],c3);plot([0 1 1 0 0],[0 0 1 1 0]);disp('W');
  "b{1}" : Constant  Value=[1.5598552654548620832741789854480884969234466552734375;-1.3302789635524174816083586847526021301746368408203125]
      mask Display: e = 0.06;c1 = [120 150 230]/255;c2 = ([120 150 230]+0)/383;c3 = ([120 150 230]+128)/383;patch([0 1 1 0],[0 0 1 1],c1);patch([0 1 1 1-e 1-e 0+e],[0 0 1 1-e 0+e 0+e],c2);patch([0 0 1 1-e 0+e 0+e],[0 1 1 1-e 1-e 0+e],c3);plot([0 1 1 0 0],[0 0 1 1 0]);disp('b');
  netsum : Sum  Inputs=2  InputSameDT=on  SaturateOnIntegerOverflow=on  OutDataTypeStr=Inherit: Same as first input
      mask Display: e = 0.06;c1 = [120 150 230]/255;c2 = ([120 150 230]+0)/383;c3 = ([120 150 230]+128)/383;patch([0 1 1 0],[0 0 1 1],c1);patch([0 1 1 1-e 1-e 0+e],[0 0 1 1-e 0+e 0+e],c2);patch([0 0 1 1-e 0+e 0+e],[0 1 1 1-e 1-e 0+e],c3);plot([0 1 1 0 0],[0 0 1 1 0]);disp('+');
  tansig : neural/Transfer Functions/tansig
  "a{1}" : Outport  InitialOutput=[0;0]
      mask Display: e = 0.06;c1 = [120 230 180]/255;c2 = ([120 230 180]+0)/(256+128);c3 = ([120 230 180]+128)/(256+128);patch([0 1 1 0],[0 0 1 1],c1);patch([0 1 1 1-e 1-e 0+e],[0 0 1 1-e 0+e 0+e],c2);patch([0 0 1 1-e 0+e 0+e],[0 1 1 1-e 1-e 0+e],c3);plot([0 1 1 0 0],[0 0 1 1 0]);
  wires:
  "p{1}"/1 -> Delays 1/1("p{1}")
  Delays 1/1("pd{1,1}") -> "IW{1,1}"/1("pd{1,1}")
  "IW{1,1}"/1("iz{1,1}") -> netsum/1
  "b{1}"/1 -> netsum/2
  netsum/1 -> tansig/1
  tansig/1 -> "a{1}"/1

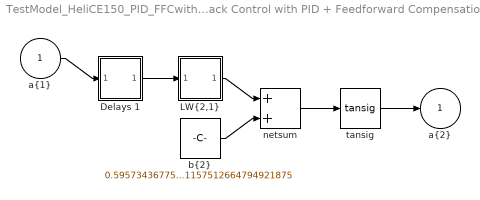
== system TestModel_HeliCE150_PID_FFCwithNN/Feedback Control with PID + Feedforward Compensation with Neural Networks/FFNet - Multi Layer Perceptron [2 1 2] Unstable region of psi: <90°,115°> In: [psi_d; phi_d] // Out: [u_1; u_2]/Layer 2 ==
  "a{1} " : Inport  PortDimensions=2
      mask Display: e = 0.06;c1 = [120 230 180]/255;c2 = ([120 230 180]+0)/(256+128);c3 = ([120 230 180]+128)/(256+128);patch([0 1 1 0],[0 0 1 1],c1);patch([0 1 1 1-e 1-e 0+e],[0 0 1 1-e 0+e 0+e],c2);patch([0 0 1 1-e 0+e 0+e],[0 1 1 1-e 1-e 0+e],c3);plot([0 1 1 0 0],[0 0 1 1 0]);
  Delays 1 : Subsystem
      mask Display: e = 0.06;c1 = [120 150 230]/255;c2 = ([120 150 230]+0)/383;c3 = ([120 150 230]+128)/383;patch([0 1 1 0],[0 0 1 1],c1);patch([0 1 1 1-e 1-e 0+e],[0 0 1 1-e 0+e 0+e],c2);patch([0 0 1 1-e 0+e 0+e],[0 1 1 1-e 1-e 0+e],c3);plot([0 1 1 0 0],[0 0 1 1 0]);disp('0');
  "LW{2,1}" : Subsystem
      mask Display: e = 0.06;c1 = [120 150 230]/255;c2 = ([120 150 230]+0)/383;c3 = ([120 150 230]+128)/383;patch([0 1 1 0],[0 0 1 1],c1);patch([0 1 1 1-e 1-e 0+e],[0 0 1 1-e 0+e 0+e],c2);patch([0 0 1 1-e 0+e 0+e],[0 1 1 1-e 1-e 0+e],c3);plot([0 1 1 0 0],[0 0 1 1 0]);disp('W');
  "b{2}" : Constant  Value=0.59573436775278032495606339580263011157512664794921875
      mask Display: e = 0.06;c1 = [120 150 230]/255;c2 = ([120 150 230]+0)/383;c3 = ([120 150 230]+128)/383;patch([0 1 1 0],[0 0 1 1],c1);patch([0 1 1 1-e 1-e 0+e],[0 0 1 1-e 0+e 0+e],c2);patch([0 0 1 1-e 0+e 0+e],[0 1 1 1-e 1-e 0+e],c3);plot([0 1 1 0 0],[0 0 1 1 0]);disp('b');
  netsum : Sum  Inputs=2  InputSameDT=on  SaturateOnIntegerOverflow=on  OutDataTypeStr=Inherit: Same as first input
      mask Display: e = 0.06;c1 = [120 150 230]/255;c2 = ([120 150 230]+0)/383;c3 = ([120 150 230]+128)/383;patch([0 1 1 0],[0 0 1 1],c1);patch([0 1 1 1-e 1-e 0+e],[0 0 1 1-e 0+e 0+e],c2);patch([0 0 1 1-e 0+e 0+e],[0 1 1 1-e 1-e 0+e],c3);plot([0 1 1 0 0],[0 0 1 1 0]);disp('+');
  tansig : neural/Transfer Functions/tansig
  "a{2}" : Outport  InitialOutput=0
      mask Display: e = 0.06;c1 = [120 230 180]/255;c2 = ([120 230 180]+0)/(256+128);c3 = ([120 230 180]+128)/(256+128);patch([0 1 1 0],[0 0 1 1],c1);patch([0 1 1 1-e 1-e 0+e],[0 0 1 1-e 0+e 0+e],c2);patch([0 0 1 1-e 0+e 0+e],[0 1 1 1-e 1-e 0+e],c3);plot([0 1 1 0 0],[0 0 1 1 0]);
  wires:
  "a{1} "/1 -> Delays 1/1("p{2}")
  Delays 1/1("pd{2,1}") -> "LW{2,1}"/1("ad{2,1}")
  "LW{2,1}"/1("lz{2,1}") -> netsum/1
  "b{2}"/1 -> netsum/2
  netsum/1 -> tansig/1
  tansig/1 -> "a{2}"/1

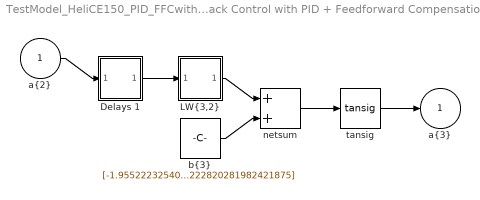
== system TestModel_HeliCE150_PID_FFCwithNN/Feedback Control with PID + Feedforward Compensation with Neural Networks/FFNet - Multi Layer Perceptron [2 1 2] Unstable region of psi: <90°,115°> In: [psi_d; phi_d] // Out: [u_1; u_2]/Layer 3 ==
  "a{2} " : Inport  PortDimensions=1
      mask Display: e = 0.06;c1 = [120 230 180]/255;c2 = ([120 230 180]+0)/(256+128);c3 = ([120 230 180]+128)/(256+128);patch([0 1 1 0],[0 0 1 1],c1);patch([0 1 1 1-e 1-e 0+e],[0 0 1 1-e 0+e 0+e],c2);patch([0 0 1 1-e 0+e 0+e],[0 1 1 1-e 1-e 0+e],c3);plot([0 1 1 0 0],[0 0 1 1 0]);
  Delays 1 : Subsystem
      mask Display: e = 0.06;c1 = [120 150 230]/255;c2 = ([120 150 230]+0)/383;c3 = ([120 150 230]+128)/383;patch([0 1 1 0],[0 0 1 1],c1);patch([0 1 1 1-e 1-e 0+e],[0 0 1 1-e 0+e 0+e],c2);patch([0 0 1 1-e 0+e 0+e],[0 1 1 1-e 1-e 0+e],c3);plot([0 1 1 0 0],[0 0 1 1 0]);disp('0');
  "LW{3,2}" : Subsystem
      mask Display: e = 0.06;c1 = [120 150 230]/255;c2 = ([120 150 230]+0)/383;c3 = ([120 150 230]+128)/383;patch([0 1 1 0],[0 0 1 1],c1);patch([0 1 1 1-e 1-e 0+e],[0 0 1 1-e 0+e 0+e],c2);patch([0 0 1 1-e 0+e 0+e],[0 1 1 1-e 1-e 0+e],c3);plot([0 1 1 0 0],[0 0 1 1 0]);disp('W');
  "b{3}" : Constant  Value=[-1.955222325409454509070883432286791503429412841796875;-3.173472597551373564073173838551156222820281982421875]
      mask Display: e = 0.06;c1 = [120 150 230]/255;c2 = ([120 150 230]+0)/383;c3 = ([120 150 230]+128)/383;patch([0 1 1 0],[0 0 1 1],c1);patch([0 1 1 1-e 1-e 0+e],[0 0 1 1-e 0+e 0+e],c2);patch([0 0 1 1-e 0+e 0+e],[0 1 1 1-e 1-e 0+e],c3);plot([0 1 1 0 0],[0 0 1 1 0]);disp('b');
  netsum : Sum  Inputs=2  InputSameDT=on  SaturateOnIntegerOverflow=on  OutDataTypeStr=Inherit: Same as first input
      mask Display: e = 0.06;c1 = [120 150 230]/255;c2 = ([120 150 230]+0)/383;c3 = ([120 150 230]+128)/383;patch([0 1 1 0],[0 0 1 1],c1);patch([0 1 1 1-e 1-e 0+e],[0 0 1 1-e 0+e 0+e],c2);patch([0 0 1 1-e 0+e 0+e],[0 1 1 1-e 1-e 0+e],c3);plot([0 1 1 0 0],[0 0 1 1 0]);disp('+');
  tansig : neural/Transfer Functions/tansig
  "a{3}" : Outport  InitialOutput=[0;0]
      mask Display: e = 0.06;c1 = [120 230 180]/255;c2 = ([120 230 180]+0)/(256+128);c3 = ([120 230 180]+128)/(256+128);patch([0 1 1 0],[0 0 1 1],c1);patch([0 1 1 1-e 1-e 0+e],[0 0 1 1-e 0+e 0+e],c2);patch([0 0 1 1-e 0+e 0+e],[0 1 1 1-e 1-e 0+e],c3);plot([0 1 1 0 0],[0 0 1 1 0]);
  wires:
  "a{2} "/1 -> Delays 1/1("p{3}")
  Delays 1/1("pd{3,2}") -> "LW{3,2}"/1("ad{3,2}")
  "LW{3,2}"/1("lz{3,2}") -> netsum/1
  "b{3}"/1 -> netsum/2
  netsum/1 -> tansig/1
  tansig/1 -> "a{3}"/1

== system TestModel_HeliCE150_PID_FFCwithNN/Feedback Control with PID + Feedforward Compensation with Neural Networks/FFNet - Multi Layer Perceptron [2 1 2] Unstable region of psi: <90°,115°> In: [psi_d; phi_d] // Out: [u_1; u_2]/Layer 4 ==
  "a{3} " : Inport  PortDimensions=2
      mask Display: e = 0.06;c1 = [120 230 180]/255;c2 = ([120 230 180]+0)/(256+128);c3 = ([120 230 180]+128)/(256+128);patch([0 1 1 0],[0 0 1 1],c1);patch([0 1 1 1-e 1-e 0+e],[0 0 1 1-e 0+e 0+e],c2);patch([0 0 1 1-e 0+e 0+e],[0 1 1 1-e 1-e 0+e],c3);plot([0 1 1 0 0],[0 0 1 1 0]);
  Delays 1 : Subsystem
      mask Display: e = 0.06;c1 = [120 150 230]/255;c2 = ([120 150 230]+0)/383;c3 = ([120 150 230]+128)/383;patch([0 1 1 0],[0 0 1 1],c1);patch([0 1 1 1-e 1-e 0+e],[0 0 1 1-e 0+e 0+e],c2);patch([0 0 1 1-e 0+e 0+e],[0 1 1 1-e 1-e 0+e],c3);plot([0 1 1 0 0],[0 0 1 1 0]);disp('0');
  "LW{4,3}" : Subsystem
      mask Display: e = 0.06;c1 = [120 150 230]/255;c2 = ([120 150 230]+0)/383;c3 = ([120 150 230]+128)/383;patch([0 1 1 0],[0 0 1 1],c1);patch([0 1 1 1-e 1-e 0+e],[0 0 1 1-e 0+e 0+e],c2);patch([0 0 1 1-e 0+e 0+e],[0 1 1 1-e 1-e 0+e],c3);plot([0 1 1 0 0],[0 0 1 1 0]);disp('W');
  "b{4}" : Constant  Value=[-0.4018107677645215147776980302296578884124755859375;0.399606614415510763560490659074275754392147064208984375]
      mask Display: e = 0.06;c1 = [120 150 230]/255;c2 = ([120 150 230]+0)/383;c3 = ([120 150 230]+128)/383;patch([0 1 1 0],[0 0 1 1],c1);patch([0 1 1 1-e 1-e 0+e],[0 0 1 1-e 0+e 0+e],c2);patch([0 0 1 1-e 0+e 0+e],[0 1 1 1-e 1-e 0+e],c3);plot([0 1 1 0 0],[0 0 1 1 0]);disp('b');
  netsum : Sum  Inputs=2  InputSameDT=on  SaturateOnIntegerOverflow=on  OutDataTypeStr=Inherit: Same as first input
      mask Display: e = 0.06;c1 = [120 150 230]/255;c2 = ([120 150 230]+0)/383;c3 = ([120 150 230]+128)/383;patch([0 1 1 0],[0 0 1 1],c1);patch([0 1 1 1-e 1-e 0+e],[0 0 1 1-e 0+e 0+e],c2);patch([0 0 1 1-e 0+e 0+e],[0 1 1 1-e 1-e 0+e],c3);plot([0 1 1 0 0],[0 0 1 1 0]);disp('+');
  purelin : neural/Transfer Functions/purelin
  "a{4}" : Outport  InitialOutput=[0;0]
      mask Display: e = 0.06;c1 = [120 230 180]/255;c2 = ([120 230 180]+0)/(256+128);c3 = ([120 230 180]+128)/(256+128);patch([0 1 1 0],[0 0 1 1],c1);patch([0 1 1 1-e 1-e 0+e],[0 0 1 1-e 0+e 0+e],c2);patch([0 0 1 1-e 0+e 0+e],[0 1 1 1-e 1-e 0+e],c3);plot([0 1 1 0 0],[0 0 1 1 0]);
  wires:
  "a{3} "/1 -> Delays 1/1("p{4}")
  Delays 1/1("pd{4,3}") -> "LW{4,3}"/1("ad{4,3}")
  "LW{4,3}"/1("lz{4,3}") -> netsum/1
  "b{4}"/1 -> netsum/2
  netsum/1 -> purelin/1
  purelin/1 -> "a{4}"/1

== system TestModel_HeliCE150_PID_FFCwithNN/Feedback Control with PID + Feedforward Compensation with Neural Networks/FFNet - Multi Layer Perceptron [2 1 2] Unstable region of psi: <90°,115°> In: [psi_d; phi_d] // Out: [u_1; u_2]/Process Input 1 ==
  x : Inport  PortDimensions=2
      mask Display: e = 0.06;c1 = [120 230 180]/255;c2 = ([120 230 180]+0)/(256+128);c3 = ([120 230 180]+128)/(256+128);patch([0 1 1 0],[0 0 1 1],c1);patch([0 1 1 1-e 1-e 0+e],[0 0 1 1-e 0+e 0+e],c2);patch([0 0 1 1-e 0+e 0+e],[0 1 1 1-e 1-e 0+e],c3);plot([0 1 1 0 0],[0 0 1 1 0]);
  mapminmax : neural/Processing Functions/mapminmax  xmin=[91.1316816411983552370656980202;-90.0672478770217139754095114768]  xmax=[113.213573919003067658195504919;90.0365841038475878121971618384]  ymin=-1  ymax=1
  p : Outport  PortDimensions=2
      mask Display: e = 0.06;c1 = [120 230 180]/255;c2 = ([120 230 180]+0)/(256+128);c3 = ([120 230 180]+128)/(256+128);patch([0 1 1 0],[0 0 1 1],c1);patch([0 1 1 1-e 1-e 0+e],[0 0 1 1-e 0+e 0+e],c2);patch([0 0 1 1-e 0+e 0+e],[0 1 1 1-e 1-e 0+e],c3);plot([0 1 1 0 0],[0 0 1 1 0]);
  wires:
  x/1 -> mapminmax/1
  mapminmax/1 -> p/1

== system TestModel_HeliCE150_PID_FFCwithNN/Feedback Control with PID + Feedforward Compensation with Neural Networks/FFNet - Multi Layer Perceptron [2 1 2] Unstable region of psi: <90°,115°> In: [psi_d; phi_d] // Out: [u_1; u_2]/Process Output 1 ==
  a : Inport  PortDimensions=2
      mask Display: e = 0.06;c1 = [120 230 180]/255;c2 = ([120 230 180]+0)/(256+128);c3 = ([120 230 180]+128)/(256+128);patch([0 1 1 0],[0 0 1 1],c1);patch([0 1 1 1-e 1-e 0+e],[0 0 1 1-e 0+e 0+e],c2);patch([0 0 1 1-e 0+e 0+e],[0 1 1 1-e 1-e 0+e],c3);plot([0 1 1 0 0],[0 0 1 1 0]);
  mapminmax_reverse : neural/Processing Functions/mapminmax_reverse  xmin=[0.527027011356937968855618237285;0.0261879450134974156583211879479]  xmax=[0.560993426727410926524441947549;0.0299887526688913733097230363001]  ymin=-1  ymax=1
  y : Outport  PortDimensions=2
      mask Display: e = 0.06;c1 = [120 230 180]/255;c2 = ([120 230 180]+0)/(256+128);c3 = ([120 230 180]+128)/(256+128);patch([0 1 1 0],[0 0 1 1],c1);patch([0 1 1 1-e 1-e 0+e],[0 0 1 1-e 0+e 0+e],c2);patch([0 0 1 1-e 0+e 0+e],[0 1 1 1-e 1-e 0+e],c3);plot([0 1 1 0 0],[0 0 1 1 0]);
  wires:
  a/1 -> mapminmax_reverse/1
  mapminmax_reverse/1 -> y/1

== system TestModel_HeliCE150_PID_FFCwithNN/Feedback Control with PID + Feedforward Compensation with Neural Networks/FFNet - Multi Layer Perceptron [2 2] In: [psi_d; phi_d] // Out: [u_1; u_2] 2/Layer 1 ==
  "p{1}" : Inport  PortDimensions=2
      mask Display: e = 0.06;c1 = [120 230 180]/255;c2 = ([120 230 180]+0)/(256+128);c3 = ([120 230 180]+128)/(256+128);patch([0 1 1 0],[0 0 1 1],c1);patch([0 1 1 1-e 1-e 0+e],[0 0 1 1-e 0+e 0+e],c2);patch([0 0 1 1-e 0+e 0+e],[0 1 1 1-e 1-e 0+e],c3);plot([0 1 1 0 0],[0 0 1 1 0]);
  Delays 1 : Subsystem
      mask Display: e = 0.06;c1 = [120 150 230]/255;c2 = ([120 150 230]+0)/383;c3 = ([120 150 230]+128)/383;patch([0 1 1 0],[0 0 1 1],c1);patch([0 1 1 1-e 1-e 0+e],[0 0 1 1-e 0+e 0+e],c2);patch([0 0 1 1-e 0+e 0+e],[0 1 1 1-e 1-e 0+e],c3);plot([0 1 1 0 0],[0 0 1 1 0]);disp('0');
  "IW{1,1}" : Subsystem
      mask Display: e = 0.06;c1 = [120 150 230]/255;c2 = ([120 150 230]+0)/383;c3 = ([120 150 230]+128)/383;patch([0 1 1 0],[0 0 1 1],c1);patch([0 1 1 1-e 1-e 0+e],[0 0 1 1-e 0+e 0+e],c2);patch([0 0 1 1-e 0+e 0+e],[0 1 1 1-e 1-e 0+e],c3);plot([0 1 1 0 0],[0 0 1 1 0]);disp('W');
  "b{1}" : Constant  Value=[0.10576736253171890866919824247815995477139949798583984375;3.414276721935223246617852055351249873638153076171875]
      mask Display: e = 0.06;c1 = [120 150 230]/255;c2 = ([120 150 230]+0)/383;c3 = ([120 150 230]+128)/383;patch([0 1 1 0],[0 0 1 1],c1);patch([0 1 1 1-e 1-e 0+e],[0 0 1 1-e 0+e 0+e],c2);patch([0 0 1 1-e 0+e 0+e],[0 1 1 1-e 1-e 0+e],c3);plot([0 1 1 0 0],[0 0 1 1 0]);disp('b');
  netsum : Sum  Inputs=2  InputSameDT=on  SaturateOnIntegerOverflow=on  OutDataTypeStr=Inherit: Same as first input
      mask Display: e = 0.06;c1 = [120 150 230]/255;c2 = ([120 150 230]+0)/383;c3 = ([120 150 230]+128)/383;patch([0 1 1 0],[0 0 1 1],c1);patch([0 1 1 1-e 1-e 0+e],[0 0 1 1-e 0+e 0+e],c2);patch([0 0 1 1-e 0+e 0+e],[0 1 1 1-e 1-e 0+e],c3);plot([0 1 1 0 0],[0 0 1 1 0]);disp('+');
  tansig : neural/Transfer Functions/tansig
  "a{1}" : Outport  InitialOutput=[0;0]
      mask Display: e = 0.06;c1 = [120 230 180]/255;c2 = ([120 230 180]+0)/(256+128);c3 = ([120 230 180]+128)/(256+128);patch([0 1 1 0],[0 0 1 1],c1);patch([0 1 1 1-e 1-e 0+e],[0 0 1 1-e 0+e 0+e],c2);patch([0 0 1 1-e 0+e 0+e],[0 1 1 1-e 1-e 0+e],c3);plot([0 1 1 0 0],[0 0 1 1 0]);
  wires:
  tansig/1 -> "a{1}"/1
  netsum/1 -> tansig/1
  "b{1}"/1 -> netsum/2
  "IW{1,1}"/1("iz{1,1}") -> netsum/1
  Delays 1/1("pd{1,1}") -> "IW{1,1}"/1("pd{1,1}")
  "p{1}"/1 -> Delays 1/1("p{1}")

== system TestModel_HeliCE150_PID_FFCwithNN/Feedback Control with PID + Feedforward Compensation with Neural Networks/FFNet - Multi Layer Perceptron [2 2] In: [psi_d; phi_d] // Out: [u_1; u_2] 2/Layer 2 ==
  "a{1} " : Inport  PortDimensions=2
      mask Display: e = 0.06;c1 = [120 230 180]/255;c2 = ([120 230 180]+0)/(256+128);c3 = ([120 230 180]+128)/(256+128);patch([0 1 1 0],[0 0 1 1],c1);patch([0 1 1 1-e 1-e 0+e],[0 0 1 1-e 0+e 0+e],c2);patch([0 0 1 1-e 0+e 0+e],[0 1 1 1-e 1-e 0+e],c3);plot([0 1 1 0 0],[0 0 1 1 0]);
  Delays 1 : Subsystem
      mask Display: e = 0.06;c1 = [120 150 230]/255;c2 = ([120 150 230]+0)/383;c3 = ([120 150 230]+128)/383;patch([0 1 1 0],[0 0 1 1],c1);patch([0 1 1 1-e 1-e 0+e],[0 0 1 1-e 0+e 0+e],c2);patch([0 0 1 1-e 0+e 0+e],[0 1 1 1-e 1-e 0+e],c3);plot([0 1 1 0 0],[0 0 1 1 0]);disp('0');
  "LW{2,1}" : Subsystem
      mask Display: e = 0.06;c1 = [120 150 230]/255;c2 = ([120 150 230]+0)/383;c3 = ([120 150 230]+128)/383;patch([0 1 1 0],[0 0 1 1],c1);patch([0 1 1 1-e 1-e 0+e],[0 0 1 1-e 0+e 0+e],c2);patch([0 0 1 1-e 0+e 0+e],[0 1 1 1-e 1-e 0+e],c3);plot([0 1 1 0 0],[0 0 1 1 0]);disp('W');
  "b{2}" : Constant  Value=[2.842198943889313600408286220044828951358795166015625;-1.695234382048245169727351822075434029102325439453125]
      mask Display: e = 0.06;c1 = [120 150 230]/255;c2 = ([120 150 230]+0)/383;c3 = ([120 150 230]+128)/383;patch([0 1 1 0],[0 0 1 1],c1);patch([0 1 1 1-e 1-e 0+e],[0 0 1 1-e 0+e 0+e],c2);patch([0 0 1 1-e 0+e 0+e],[0 1 1 1-e 1-e 0+e],c3);plot([0 1 1 0 0],[0 0 1 1 0]);disp('b');
  netsum : Sum  Inputs=2  InputSameDT=on  SaturateOnIntegerOverflow=on  OutDataTypeStr=Inherit: Same as first input
      mask Display: e = 0.06;c1 = [120 150 230]/255;c2 = ([120 150 230]+0)/383;c3 = ([120 150 230]+128)/383;patch([0 1 1 0],[0 0 1 1],c1);patch([0 1 1 1-e 1-e 0+e],[0 0 1 1-e 0+e 0+e],c2);patch([0 0 1 1-e 0+e 0+e],[0 1 1 1-e 1-e 0+e],c3);plot([0 1 1 0 0],[0 0 1 1 0]);disp('+');
  tansig : neural/Transfer Functions/tansig
  "a{2}" : Outport  InitialOutput=[0;0]
      mask Display: e = 0.06;c1 = [120 230 180]/255;c2 = ([120 230 180]+0)/(256+128);c3 = ([120 230 180]+128)/(256+128);patch([0 1 1 0],[0 0 1 1],c1);patch([0 1 1 1-e 1-e 0+e],[0 0 1 1-e 0+e 0+e],c2);patch([0 0 1 1-e 0+e 0+e],[0 1 1 1-e 1-e 0+e],c3);plot([0 1 1 0 0],[0 0 1 1 0]);
  wires:
  tansig/1 -> "a{2}"/1
  netsum/1 -> tansig/1
  "b{2}"/1 -> netsum/2
  "LW{2,1}"/1("lz{2,1}") -> netsum/1
  Delays 1/1("pd{2,1}") -> "LW{2,1}"/1("ad{2,1}")
  "a{1} "/1 -> Delays 1/1("p{2}")

== system TestModel_HeliCE150_PID_FFCwithNN/Feedback Control with PID + Feedforward Compensation with Neural Networks/FFNet - Multi Layer Perceptron [2 2] In: [psi_d; phi_d] // Out: [u_1; u_2] 2/Layer 3 ==
  "a{2} " : Inport  PortDimensions=2
      mask Display: e = 0.06;c1 = [120 230 180]/255;c2 = ([120 230 180]+0)/(256+128);c3 = ([120 230 180]+128)/(256+128);patch([0 1 1 0],[0 0 1 1],c1);patch([0 1 1 1-e 1-e 0+e],[0 0 1 1-e 0+e 0+e],c2);patch([0 0 1 1-e 0+e 0+e],[0 1 1 1-e 1-e 0+e],c3);plot([0 1 1 0 0],[0 0 1 1 0]);
  Delays 1 : Subsystem
      mask Display: e = 0.06;c1 = [120 150 230]/255;c2 = ([120 150 230]+0)/383;c3 = ([120 150 230]+128)/383;patch([0 1 1 0],[0 0 1 1],c1);patch([0 1 1 1-e 1-e 0+e],[0 0 1 1-e 0+e 0+e],c2);patch([0 0 1 1-e 0+e 0+e],[0 1 1 1-e 1-e 0+e],c3);plot([0 1 1 0 0],[0 0 1 1 0]);disp('0');
  "LW{3,2}" : Subsystem
      mask Display: e = 0.06;c1 = [120 150 230]/255;c2 = ([120 150 230]+0)/383;c3 = ([120 150 230]+128)/383;patch([0 1 1 0],[0 0 1 1],c1);patch([0 1 1 1-e 1-e 0+e],[0 0 1 1-e 0+e 0+e],c2);patch([0 0 1 1-e 0+e 0+e],[0 1 1 1-e 1-e 0+e],c3);plot([0 1 1 0 0],[0 0 1 1 0]);disp('W');
  "b{3}" : Constant  Value=[-3.57071060797095807259893263108097016811370849609375;-3.722542157898581560715456362231634557247161865234375]
      mask Display: e = 0.06;c1 = [120 150 230]/255;c2 = ([120 150 230]+0)/383;c3 = ([120 150 230]+128)/383;patch([0 1 1 0],[0 0 1 1],c1);patch([0 1 1 1-e 1-e 0+e],[0 0 1 1-e 0+e 0+e],c2);patch([0 0 1 1-e 0+e 0+e],[0 1 1 1-e 1-e 0+e],c3);plot([0 1 1 0 0],[0 0 1 1 0]);disp('b');
  netsum : Sum  Inputs=2  InputSameDT=on  SaturateOnIntegerOverflow=on  OutDataTypeStr=Inherit: Same as first input
      mask Display: e = 0.06;c1 = [120 150 230]/255;c2 = ([120 150 230]+0)/383;c3 = ([120 150 230]+128)/383;patch([0 1 1 0],[0 0 1 1],c1);patch([0 1 1 1-e 1-e 0+e],[0 0 1 1-e 0+e 0+e],c2);patch([0 0 1 1-e 0+e 0+e],[0 1 1 1-e 1-e 0+e],c3);plot([0 1 1 0 0],[0 0 1 1 0]);disp('+');
  purelin : neural/Transfer Functions/purelin
  "a{3}" : Outport  InitialOutput=[0;0]
      mask Display: e = 0.06;c1 = [120 230 180]/255;c2 = ([120 230 180]+0)/(256+128);c3 = ([120 230 180]+128)/(256+128);patch([0 1 1 0],[0 0 1 1],c1);patch([0 1 1 1-e 1-e 0+e],[0 0 1 1-e 0+e 0+e],c2);patch([0 0 1 1-e 0+e 0+e],[0 1 1 1-e 1-e 0+e],c3);plot([0 1 1 0 0],[0 0 1 1 0]);
  wires:
  purelin/1 -> "a{3}"/1
  netsum/1 -> purelin/1
  "b{3}"/1 -> netsum/2
  "LW{3,2}"/1("lz{3,2}") -> netsum/1
  Delays 1/1("pd{3,2}") -> "LW{3,2}"/1("ad{3,2}")
  "a{2} "/1 -> Delays 1/1("p{3}")
